simulink model "rc_update"  (R2024b)
settings: Solver=FixedStepAuto  StartTime=0.0  StopTime=10.0  FixedStep=0.005  RelTol=1e-3
undefined symbols (not defined in the file): MANUAL_CONTROL_SETPOINT, RC10_DZ, RC10_MAX, RC10_MIN, RC10_REV, RC10_TRIM, RC11_DZ, RC11_MAX, RC11_MIN, RC11_REV, RC11_TRIM, RC12_DZ, RC12_MAX, RC12_MIN, RC12_REV, RC12_TRIM, RC13_DZ, RC13_MAX, RC13_MIN, RC13_REV, RC13_TRIM, RC14_DZ, RC14_MAX, RC14_MIN, RC14_REV, RC14_TRIM, RC15_DZ, RC15_MAX, RC15_MIN, RC15_REV, RC15_TRIM, RC16_DZ, RC16_MAX, RC16_MIN, RC16_REV, RC16_TRIM, RC17_DZ, RC17_MAX, RC17_MIN, RC17_REV, RC17_TRIM, RC18_DZ, RC18_MAX, RC18_MIN, RC18_REV, RC18_TRIM, RC1_DZ, RC1_MAX, RC1_MIN, RC1_REV, RC1_TRIM, RC2_DZ, RC2_MAX, RC2_MIN, RC2_REV, RC2_TRIM, RC3_DZ, RC3_MAX, RC3_MIN, RC3_REV ... (+71)
libraries: simulink x1
settings Model: DataDictionary=nextpilot_datadict.sldd  Creator=DELL  LastModifiedBy=93114
settings OptimizationCC: DefaultUnderspecifiedDataType=single
settings DebuggingCC: UnconnectedInputMsg=warning  UnconnectedOutputMsg=warning  UnconnectedLineMsg=warning
settings ModelReferenceCC: EnableRefExpFcnMdlSchedulingChecks=on
settings RTWCC: GPUComputeCapability=3.5  DLArmComputeVersion=19.05

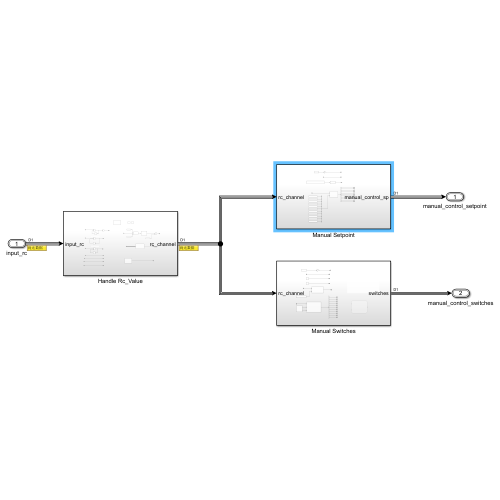
[thumbnail: Simulink's stored preview of the top-level diagram]
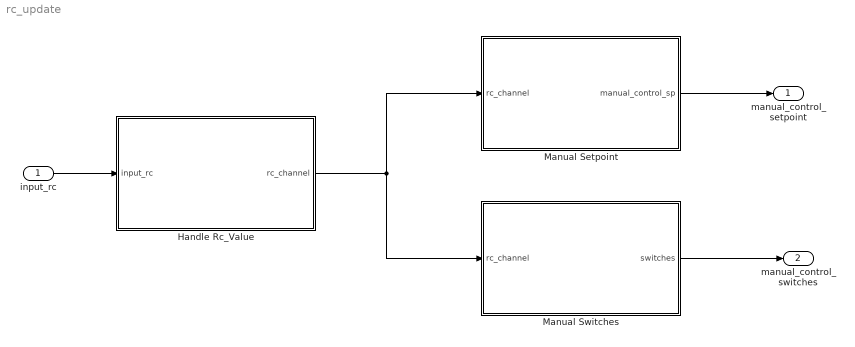
== system rc_update ==
  input_rc : Inport  OutDataTypeStr=Bus: input_rc_s
  Handle Rc_Value : Subsystem
  Manual Setpoint : Subsystem
  Manual Switches : Subsystem
  manual_control_setpoint : Outport  OutDataTypeStr=Bus: manual_control_setpoint_s
  manual_control_switches : Outport  Port=2  OutDataTypeStr=Bus: manual_control_switches_s
  wires:
  input_rc/1 -> Handle Rc_Value/1(input_rc)
  Handle Rc_Value/1(rc_channel) -> Manual Setpoint/1(rc_channel), Manual Switches/1(rc_channel)
  Manual Setpoint/1(manual_control_sp) -> manual_control_setpoint/1
  Manual Switches/1(switches) -> manual_control_switches/1

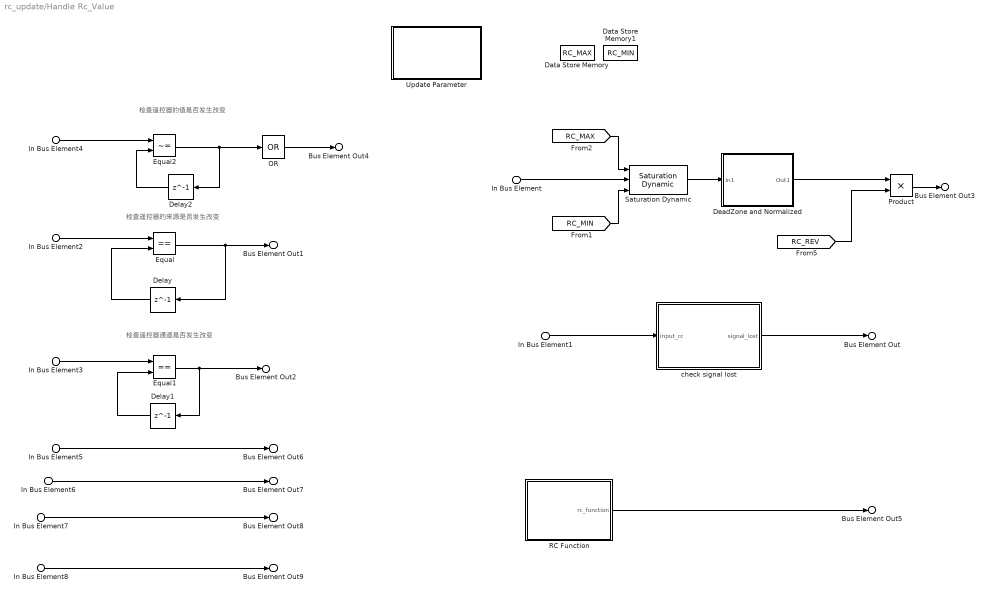
== system rc_update/Handle Rc_Value ==
  note: 检查遥控器通道是否发生改变
  note: 检查遥控器的来源是否发生改变
  note: 检查遥控器的值是否发生改变
  In Bus Element1 : Inport  PortName=input_rc
  In Bus Element : Inport  PortName=input_rc  Element=values
  In Bus Element4 : Inport  PortName=input_rc  Element=values
  In Bus Element2 : Inport  PortName=input_rc  Element=input_source
  In Bus Element3 : Inport  PortName=input_rc  Element=channel_count
  In Bus Element5 : Inport  PortName=input_rc  Element=channel_count
  In Bus Element6 : Inport  PortName=input_rc  Element=rssi
  In Bus Element7 : Inport  PortName=input_rc  Element=timestamp_last_signal
  In Bus Element8 : Inport  PortName=input_rc  Element=rc_lost_frame_count
  Data Store Memory : DataStoreMemory  DataStoreName=RC_MAX  WriteAfterWriteMsg=warning  ShowAdditionalParam=off  OutDataTypeStr=single  Dimensions=18
  Data Store Memory1 : DataStoreMemory  DataStoreName=RC_MIN  WriteAfterWriteMsg=warning  ShowAdditionalParam=off  OutDataTypeStr=single  Dimensions=18
  DeadZone and Normalized : Subsystem
  Delay : Delay  DelayLength=1
  Delay1 : Delay  DelayLength=1
  Delay2 : Delay  DelayLength=1
  Equal : RelationalOperator  Operator===  OutDataTypeStr=boolean  RndMeth=Simplest  InputSameDT=off
  Equal1 : RelationalOperator  Operator===  OutDataTypeStr=boolean  RndMeth=Simplest  InputSameDT=off
  Equal2 : RelationalOperator  Operator=~=  OutDataTypeStr=boolean  RndMeth=Simplest  InputSameDT=off
  OR : Logic  Operator=OR  Inputs=1  IconShape=distinctive  AllPortsSameDT=off  OutDataTypeStr=boolean
  Product : Product
  RC Function : Subsystem
  Saturation Dynamic : simulink/Discontinuities/Saturation Dynamic  OutMin=[]  OutMax=[]  OutDataTypeStr=Inherit: Same as second input  OutDataType=fixdt(1, 16)  OutScaling=2^-10  DoSatur=off
  Update Parameter : Subsystem
  check signal lost : Stateflow chart  TreatAsAtomicUnit=on
  Bus Element Out8 : Outport  PortName=rc_channel  Element=timestamp
  Bus Element Out3 : Outport  PortName=rc_channel  Element=channels
  Bus Element Out6 : Outport  PortName=rc_channel  Element=channel_count
  Bus Element Out5 : Outport  PortName=rc_channel  Element=function
  Bus Element Out7 : Outport  PortName=rc_channel  Element=rssi
  Bus Element Out : Outport  PortName=rc_channel  Element=signal_lost
  Bus Element Out9 : Outport  PortName=rc_channel  Element=frame_drop_count
  Bus Element Out1 : Outport  PortName=rc_channel  Element=input_source_stable
  Bus Element Out2 : Outport  PortName=rc_channel  Element=channel_count_stable
  Bus Element Out4 : Outport  PortName=rc_channel  Element=rc_updated
  wires:
  [RC_REV] -> Product/2
  Saturation Dynamic/1 -> DeadZone and Normalized/1(In1)
  DeadZone and Normalized/1(Out1) -> Product/1
  [RC_MAX] -> Saturation Dynamic/1
  [RC_MIN] -> Saturation Dynamic/3
  In Bus Element/1 -> Saturation Dynamic/2
  Product/1 -> Bus Element Out3/1
  In Bus Element1/1 -> check signal lost/1(input_rc)
  check signal lost/1(signal_lost) -> Bus Element Out/1
  In Bus Element2/1 -> Equal/1
  Equal/1 -> Bus Element Out1/1, Delay/1
  Delay/1 -> Equal/2
  In Bus Element3/1 -> Equal1/1
  Equal1/1 -> Bus Element Out2/1, Delay1/1
  Delay1/1 -> Equal1/2
  In Bus Element4/1 -> Equal2/1
  Equal2/1 -> OR/1, Delay2/1
  Delay2/1 -> Equal2/2
  OR/1 -> Bus Element Out4/1
  RC Function/1(rc_function) -> Bus Element Out5/1
  In Bus Element5/1 -> Bus Element Out6/1
  In Bus Element6/1 -> Bus Element Out7/1
  In Bus Element7/1 -> Bus Element Out8/1
  In Bus Element8/1 -> Bus Element Out9/1

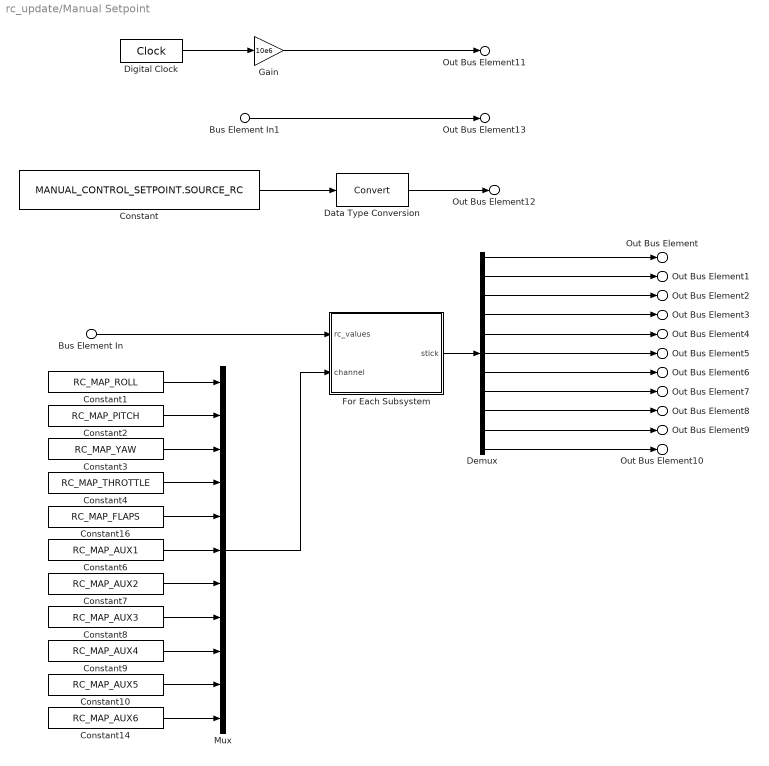
== system rc_update/Manual Setpoint ==
  Bus Element In : Inport  PortName=rc_channel  Element=channels
  Bus Element In1 : Inport  PortName=rc_channel  Element=timestamp
  Constant : Constant  Value=MANUAL_CONTROL_SETPOINT.SOURCE_RC
  Constant1 : Constant  Value=RC_MAP_ROLL
  Constant10 : Constant  Value=RC_MAP_AUX5
  Constant14 : Constant  Value=RC_MAP_AUX6
  Constant16 : Constant  Value=RC_MAP_FLAPS
  Constant2 : Constant  Value=RC_MAP_PITCH
  Constant3 : Constant  Value=RC_MAP_YAW
  Constant4 : Constant  Value=RC_MAP_THROTTLE
  Constant6 : Constant  Value=RC_MAP_AUX1
  Constant7 : Constant  Value=RC_MAP_AUX2
  Constant8 : Constant  Value=RC_MAP_AUX3
  Constant9 : Constant  Value=RC_MAP_AUX4
  Data Type Conversion : DataTypeConversion  SaturateOnIntegerOverflow=off  RndMeth=Floor
  Demux : Demux  Outputs=11.
  Digital Clock : DigitalClock  SampleTime=-1
  For Each Subsystem : Subsystem  TreatAsAtomicUnit=on
  Gain : Gain  Gain=10e6  OutDataTypeStr=uint64
  Mux : Mux  Inputs=11
  Out Bus Element11 : Outport  PortName=manual_control_sp  Element=timestamp
  Out Bus Element13 : Outport  PortName=manual_control_sp  Element=timestamp_sample
  Out Bus Element12 : Outport  PortName=manual_control_sp  Element=data_source
  Out Bus Element1 : Outport  PortName=manual_control_sp  Element=x
  Out Bus Element : Outport  PortName=manual_control_sp  Element=y
  Out Bus Element3 : Outport  PortName=manual_control_sp  Element=z
  Out Bus Element2 : Outport  PortName=manual_control_sp  Element=r
  Out Bus Element4 : Outport  PortName=manual_control_sp  Element=flaps
  Out Bus Element5 : Outport  PortName=manual_control_sp  Element=aux1
  Out Bus Element6 : Outport  PortName=manual_control_sp  Element=aux2
  Out Bus Element7 : Outport  PortName=manual_control_sp  Element=aux3
  Out Bus Element8 : Outport  PortName=manual_control_sp  Element=aux4
  Out Bus Element9 : Outport  PortName=manual_control_sp  Element=aux5
  Out Bus Element10 : Outport  PortName=manual_control_sp  Element=aux6
  wires:
  Digital Clock/1 -> Gain/1
  Constant/1 -> Data Type Conversion/1
  Bus Element In1/1 -> Out Bus Element13/1
  Gain/1 -> Out Bus Element11/1
  Data Type Conversion/1 -> Out Bus Element12/1
  Bus Element In/1 -> For Each Subsystem/1(rc_values)
  Constant1/1 -> Mux/1
  Constant2/1 -> Mux/2
  Constant4/1 -> Mux/4
  Constant3/1 -> Mux/3
  Mux/1 -> For Each Subsystem/2(channel)
  For Each Subsystem/1(stick) -> Demux/1
  Demux/5 -> Out Bus Element4/1
  Demux/4 -> Out Bus Element3/1
  Demux/6 -> Out Bus Element5/1
  Demux/3 -> Out Bus Element2/1
  Demux/7 -> Out Bus Element6/1
  Demux/2 -> Out Bus Element1/1
  Demux/8 -> Out Bus Element7/1
  Demux/1 -> Out Bus Element/1
  Demux/9 -> Out Bus Element8/1
  Demux/10 -> Out Bus Element9/1
  Demux/11 -> Out Bus Element10/1
  Constant16/1 -> Mux/5
  Constant6/1 -> Mux/6
  Constant7/1 -> Mux/7
  Constant8/1 -> Mux/8
  Constant9/1 -> Mux/9
  Constant10/1 -> Mux/10
  Constant14/1 -> Mux/11

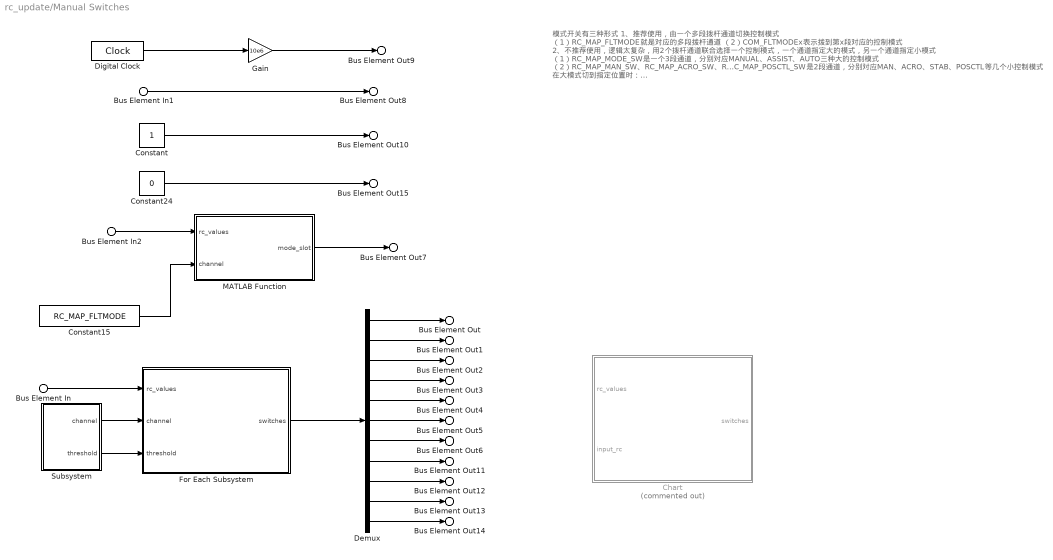
== system rc_update/Manual Switches ==
  note: 模式开关有三种形式
      |
      | 1、推荐使用，由一个多段拨杆通道切换控制模式
      | （1）RC_MAP_FLTMODE就是对应的多段拨杆通道
      | （2）COM_FLTMODEx表示拨到第x段对应的控制模式
      |
      | 2、不推荐使用，逻辑太复杂，用2个拨杆通道联合选择一个控制模式，一个通道指定大的模式，另一个通道指定小模式
      | （1）RC_MAP_MODE_SW是一个3段通道，分别对应MANUAL、ASSIST、AUTO三种大的控制模式
      | （2）RC_MAP_MAN_SW、RC_MAP_ACRO_SW、RC_MAP_STAB_SW、RC_MAP_POSCTL_SW是2段通道，分别对应MAN、ACRO、STAB、POSCTL等几个小控制模式
      |
      | 在大模式切到指定位置时：
      | （1）MANUAL模式时，优先顺序RC_MAP_MAN_SW、RC_MAP_ACRO_SW、RC_MAP_STAB_SW
      | （2）ASSIST模式时，先判断RC_MAP_POSCTL_SW通道是否打开，打开则切POSCTL，没有则切ALTCTL模式
      | （3）AUTO模式时，直接切换MISSION模式
      |
      | 3、不推荐使用，用1个按钮开关表示一个模式，长按这个按钮则切换到这个模式，
      | （1）RC_MAP_FLTM_BTN中bit位为1表示该通道作为模式按钮
      | （2）COMx_FLTMODEx表示第x个通道对应的控制模式
  Bus Element In : Inport  PortName=rc_channel  Element=channels
  Bus Element In2 : Inport  PortName=rc_channel  Element=channels
  Bus Element In1 : Inport  PortName=rc_channel  Element=timestamp
  Chart : Stateflow chart  Commented=on  TreatAsAtomicUnit=on
  Constant : Constant  OutDataTypeStr=uint32
  Constant15 : Constant  Value=RC_MAP_FLTMODE  OutDataTypeStr=single
  Constant24 : Constant  Value=0  OutDataTypeStr=uint8
  Demux : Demux  Outputs=11
  Digital Clock : DigitalClock  SampleTime=-1
  For Each Subsystem : Subsystem  TreatAsAtomicUnit=on
  Gain : Gain  Gain=10e6  OutDataTypeStr=uint64
  MATLAB Function : MATLAB Function  TreatAsAtomicUnit=on
  Subsystem : Subsystem
  Bus Element Out9 : Outport  PortName=switches  Element=timestamp
  Bus Element Out8 : Outport  PortName=switches  Element=timestamp_sample
  Bus Element Out7 : Outport  PortName=switches  Element=mode_slot
  Bus Element Out4 : Outport  PortName=switches  Element=arm_switch
  Bus Element Out : Outport  PortName=switches  Element=return_switch
  Bus Element Out1 : Outport  PortName=switches  Element=loiter_switch
  Bus Element Out2 : Outport  PortName=switches  Element=offboard_switch
  Bus Element Out3 : Outport  PortName=switches  Element=kill_switch
  Bus Element Out6 : Outport  PortName=switches  Element=gear_switch
  Bus Element Out5 : Outport  PortName=switches  Element=transition_switch
  Bus Element Out15 : Outport  PortName=switches  Element=mode_switch
  Bus Element Out11 : Outport  PortName=switches  Element=man_switch
  Bus Element Out12 : Outport  PortName=switches  Element=acro_switch
  Bus Element Out13 : Outport  PortName=switches  Element=stab_switch
  Bus Element Out14 : Outport  PortName=switches  Element=posctl_switch
  Bus Element Out10 : Outport  PortName=switches  Element=switch_changes
  wires:
  Demux/1 -> Bus Element Out/1
  Demux/2 -> Bus Element Out1/1
  Demux/3 -> Bus Element Out2/1
  Demux/4 -> Bus Element Out3/1
  Demux/5 -> Bus Element Out4/1
  Demux/6 -> Bus Element Out5/1
  Demux/7 -> Bus Element Out6/1
  Constant15/1 -> MATLAB Function/2(channel)
  Bus Element In2/1 -> MATLAB Function/1(rc_values)
  MATLAB Function/1(mode_slot) -> Bus Element Out7/1
  Bus Element In1/1 -> Bus Element Out8/1
  Gain/1 -> Bus Element Out9/1
  Digital Clock/1 -> Gain/1
  Constant/1 -> Bus Element Out10/1
  For Each Subsystem/1(switches) -> Demux/1
  Demux/8 -> Bus Element Out11/1
  Demux/9 -> Bus Element Out12/1
  Demux/10 -> Bus Element Out13/1
  Demux/11 -> Bus Element Out14/1
  Constant24/1 -> Bus Element Out15/1
  Bus Element In/1 -> For Each Subsystem/1(rc_values)
  Subsystem/1(channel) -> For Each Subsystem/2(channel)
  Subsystem/2(threshold) -> For Each Subsystem/3(threshold)

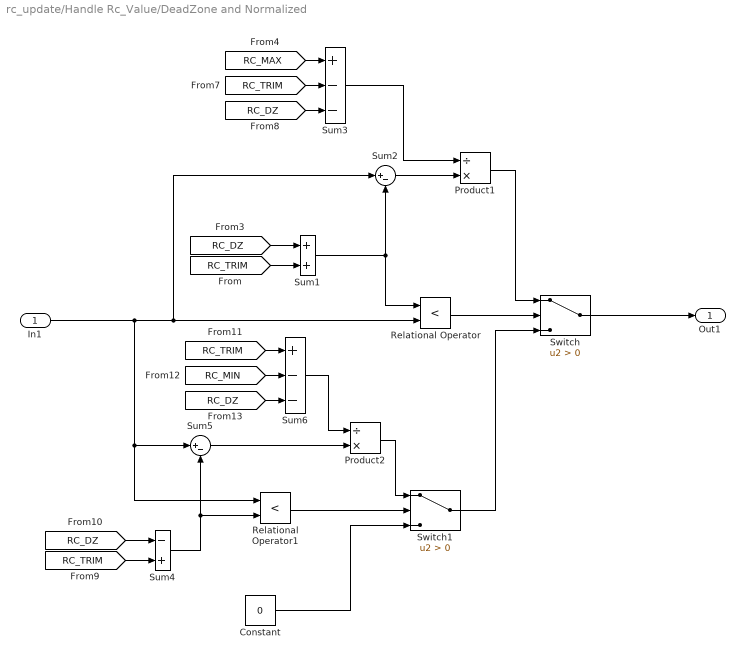
== system rc_update/Handle Rc_Value/DeadZone and Normalized ==
  In1 : Inport
  Constant : Constant  Value=0  OutDataTypeStr=single
  Product1 : Product  Inputs=/*
  Product2 : Product  Inputs=/*
  Relational Operator : RelationalOperator  Operator=<  OutDataTypeStr=boolean  RndMeth=Simplest  InputSameDT=off
  Relational Operator1 : RelationalOperator  Operator=<  OutDataTypeStr=boolean  RndMeth=Simplest  InputSameDT=off
  Sum1 : Sum  Inputs=2
  Sum2 : Sum  Inputs=|+-
  Sum3 : Sum  Inputs=+--
  Sum4 : Sum  Inputs=-+
  Sum5 : Sum  Inputs=|+-
  Sum6 : Sum  Inputs=+--
  Switch : Switch  Criteria=u2 > Threshold  SaturateOnIntegerOverflow=off  InputSameDT=off
  Switch1 : Switch  Criteria=u2 > Threshold  SaturateOnIntegerOverflow=off  InputSameDT=off
  Out1 : Outport
  wires:
  [RC_MAX] -> Sum3/1
  Sum3/1 -> Product1/1
  Product2/1 -> Switch1/1
  [RC_TRIM] -> Sum1/2
  [RC_DZ] -> Sum6/3
  Sum1/1 -> Relational Operator/1, Sum2/2
  [RC_TRIM] -> Sum3/2
  Relational Operator1/1 -> Switch1/2
  In1/1 -> Sum5/1, Relational Operator1/1, Sum2/1, Relational Operator/2
  Sum5/1 -> Product2/2
  Sum4/1 -> Sum5/2, Relational Operator1/2
  [RC_DZ] -> Sum3/3
  [RC_DZ] -> Sum1/1
  Sum2/1 -> Product1/2
  [RC_DZ] -> Sum4/1
  [RC_TRIM] -> Sum4/2
  Switch1/1 -> Switch/3
  Constant/1 -> Switch1/3
  [RC_MIN] -> Sum6/2
  Sum6/1 -> Product2/1
  Product1/1 -> Switch/1
  Relational Operator/1 -> Switch/2
  [RC_TRIM] -> Sum6/1
  Switch/1 -> Out1/1

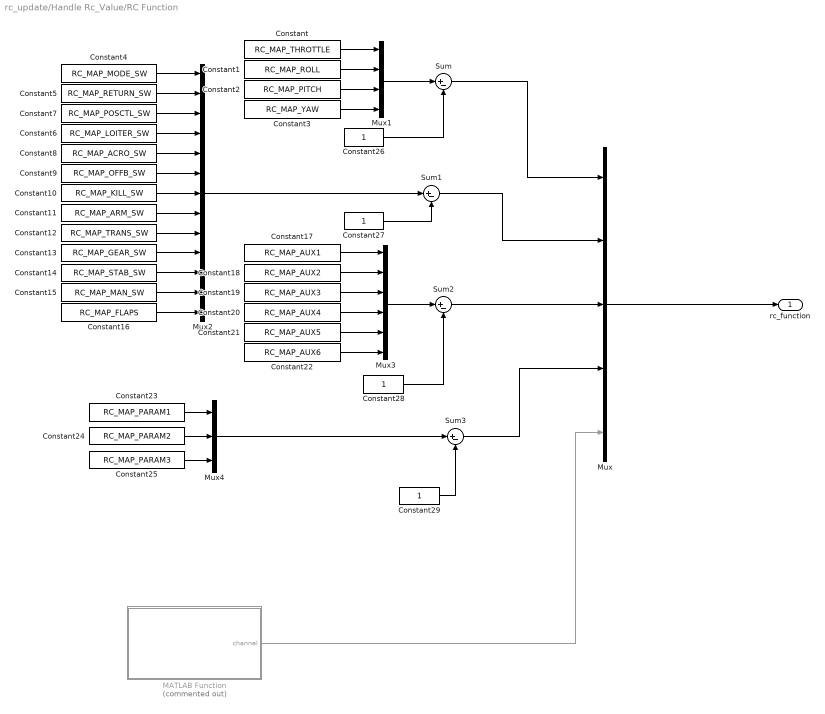
== system rc_update/Handle Rc_Value/RC Function ==
  Constant : Constant  Value=RC_MAP_THROTTLE
  Constant1 : Constant  Value=RC_MAP_ROLL
  Constant10 : Constant  Value=RC_MAP_KILL_SW
  Constant11 : Constant  Value=RC_MAP_ARM_SW
  Constant12 : Constant  Value=RC_MAP_TRANS_SW
  Constant13 : Constant  Value=RC_MAP_GEAR_SW
  Constant14 : Constant  Value=RC_MAP_STAB_SW
  Constant15 : Constant  Value=RC_MAP_MAN_SW
  Constant16 : Constant  Value=RC_MAP_FLAPS
  Constant17 : Constant  Value=RC_MAP_AUX1
  Constant18 : Constant  Value=RC_MAP_AUX2
  Constant19 : Constant  Value=RC_MAP_AUX3
  Constant2 : Constant  Value=RC_MAP_PITCH
  Constant20 : Constant  Value=RC_MAP_AUX4
  Constant21 : Constant  Value=RC_MAP_AUX5
  Constant22 : Constant  Value=RC_MAP_AUX6
  Constant23 : Constant  Value=RC_MAP_PARAM1
  Constant24 : Constant  Value=RC_MAP_PARAM2
  Constant25 : Constant  Value=RC_MAP_PARAM3
  Constant{26..29} (4 alike) : Constant  OutDataTypeStr=int8
  Constant3 : Constant  Value=RC_MAP_YAW
  Constant4 : Constant  Value=RC_MAP_MODE_SW
  Constant5 : Constant  Value=RC_MAP_RETURN_SW
  Constant6 : Constant  Value=RC_MAP_LOITER_SW
  Constant7 : Constant  Value=RC_MAP_POSCTL_SW
  Constant8 : Constant  Value=RC_MAP_ACRO_SW
  Constant9 : Constant  Value=RC_MAP_OFFB_SW
  MATLAB Function : MATLAB Function  Commented=on  TreatAsAtomicUnit=on
  Mux : Mux  Inputs=5
  Mux1 : Mux
  Mux2 : Mux  Inputs=13
  Mux3 : Mux  Inputs=6
  Mux4 : Mux  Inputs=3
  Sum{,1..3} (4 alike) : Sum  Inputs=|+-  OutDataTypeStr=int8
  rc_function : Outport
  wires:
  Mux/1 -> rc_function/1
  Constant2/1 -> Mux1/3
  Constant1/1 -> Mux1/2
  Constant/1 -> Mux1/1
  Constant3/1 -> Mux1/4
  Constant4/1 -> Mux2/1
  Constant5/1 -> Mux2/2
  Constant7/1 -> Mux2/3
  Constant6/1 -> Mux2/4
  Constant11/1 -> Mux2/8
  Constant12/1 -> Mux2/9
  Constant13/1 -> Mux2/10
  Constant14/1 -> Mux2/11
  Constant15/1 -> Mux2/12
  Constant16/1 -> Mux2/13
  Constant8/1 -> Mux2/5
  Constant9/1 -> Mux2/6
  Constant10/1 -> Mux2/7
  Constant17/1 -> Mux3/1
  Constant18/1 -> Mux3/2
  Constant19/1 -> Mux3/3
  Constant20/1 -> Mux3/4
  Constant21/1 -> Mux3/5
  Constant22/1 -> Mux3/6
  Constant23/1 -> Mux4/1
  Constant24/1 -> Mux4/2
  Constant25/1 -> Mux4/3
  Mux4/1 -> Sum3/1
  MATLAB Function/1(channel) -> Mux/5
  Mux1/1 -> Sum/1
  Sum/1 -> Mux/1
  Constant26/1 -> Sum/2
  Mux2/1 -> Sum1/1
  Constant27/1 -> Sum1/2
  Sum1/1 -> Mux/2
  Mux3/1 -> Sum2/1
  Sum2/1 -> Mux/3
  Constant28/1 -> Sum2/2
  Constant29/1 -> Sum3/2
  Sum3/1 -> Mux/4

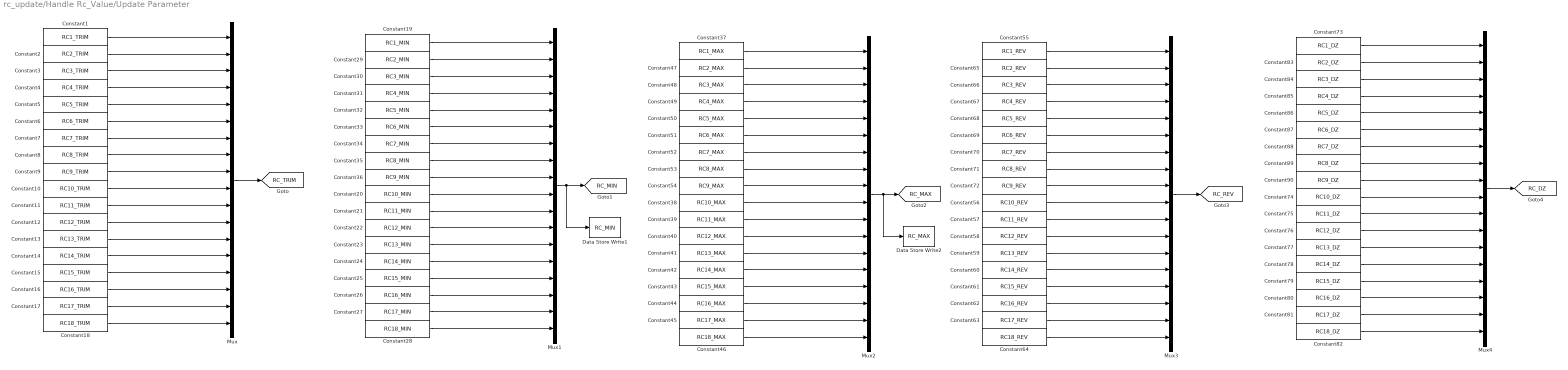
== system rc_update/Handle Rc_Value/Update Parameter ==
  Constant1 : Constant  Value=RC1_TRIM
  Constant10 : Constant  Value=RC10_TRIM
  Constant11 : Constant  Value=RC11_TRIM
  Constant12 : Constant  Value=RC12_TRIM
  Constant13 : Constant  Value=RC13_TRIM
  Constant14 : Constant  Value=RC14_TRIM
  Constant15 : Constant  Value=RC15_TRIM
  Constant16 : Constant  Value=RC16_TRIM
  Constant17 : Constant  Value=RC17_TRIM
  Constant18 : Constant  Value=RC18_TRIM
  Constant19 : Constant  Value=RC1_MIN
  Constant2 : Constant  Value=RC2_TRIM
  Constant20 : Constant  Value=RC10_MIN
  Constant21 : Constant  Value=RC11_MIN
  Constant22 : Constant  Value=RC12_MIN
  Constant23 : Constant  Value=RC13_MIN
  Constant24 : Constant  Value=RC14_MIN
  Constant25 : Constant  Value=RC15_MIN
  Constant26 : Constant  Value=RC16_MIN
  Constant27 : Constant  Value=RC17_MIN
  Constant28 : Constant  Value=RC18_MIN
  Constant29 : Constant  Value=RC2_MIN
  Constant3 : Constant  Value=RC3_TRIM
  Constant30 : Constant  Value=RC3_MIN
  Constant31 : Constant  Value=RC4_MIN
  Constant32 : Constant  Value=RC5_MIN
  Constant33 : Constant  Value=RC6_MIN
  Constant34 : Constant  Value=RC7_MIN
  Constant35 : Constant  Value=RC8_MIN
  Constant36 : Constant  Value=RC9_MIN
  Constant37 : Constant  Value=RC1_MAX
  Constant38 : Constant  Value=RC10_MAX
  Constant39 : Constant  Value=RC11_MAX
  Constant4 : Constant  Value=RC4_TRIM
  Constant40 : Constant  Value=RC12_MAX
  Constant41 : Constant  Value=RC13_MAX
  Constant42 : Constant  Value=RC14_MAX
  Constant43 : Constant  Value=RC15_MAX
  Constant44 : Constant  Value=RC16_MAX
  Constant45 : Constant  Value=RC17_MAX
  Constant46 : Constant  Value=RC18_MAX
  Constant47 : Constant  Value=RC2_MAX
  Constant48 : Constant  Value=RC3_MAX
  Constant49 : Constant  Value=RC4_MAX
  Constant5 : Constant  Value=RC5_TRIM
  Constant50 : Constant  Value=RC5_MAX
  Constant51 : Constant  Value=RC6_MAX
  Constant52 : Constant  Value=RC7_MAX
  Constant53 : Constant  Value=RC8_MAX
  Constant54 : Constant  Value=RC9_MAX
  Constant55 : Constant  Value=RC1_REV
  Constant56 : Constant  Value=RC10_REV
  Constant57 : Constant  Value=RC11_REV
  Constant58 : Constant  Value=RC12_REV
  Constant59 : Constant  Value=RC13_REV
  Constant6 : Constant  Value=RC6_TRIM
  Constant60 : Constant  Value=RC14_REV
  Constant61 : Constant  Value=RC15_REV
  Constant62 : Constant  Value=RC16_REV
  Constant63 : Constant  Value=RC17_REV
  Constant64 : Constant  Value=RC18_REV
  Constant65 : Constant  Value=RC2_REV
  Constant66 : Constant  Value=RC3_REV
  Constant67 : Constant  Value=RC4_REV
  Constant68 : Constant  Value=RC5_REV
  Constant69 : Constant  Value=RC6_REV
  Constant7 : Constant  Value=RC7_TRIM
  Constant70 : Constant  Value=RC7_REV
  Constant71 : Constant  Value=RC8_REV
  Constant72 : Constant  Value=RC9_REV
  Constant73 : Constant  Value=RC1_DZ
  Constant74 : Constant  Value=RC10_DZ
  Constant75 : Constant  Value=RC11_DZ
  Constant76 : Constant  Value=RC12_DZ
  Constant77 : Constant  Value=RC13_DZ
  Constant78 : Constant  Value=RC14_DZ
  Constant79 : Constant  Value=RC15_DZ
  Constant8 : Constant  Value=RC8_TRIM
  Constant80 : Constant  Value=RC16_DZ
  Constant81 : Constant  Value=RC17_DZ
  Constant82 : Constant  Value=RC18_DZ
  Constant83 : Constant  Value=RC2_DZ
  Constant84 : Constant  Value=RC3_DZ
  Constant85 : Constant  Value=RC4_DZ
  Constant86 : Constant  Value=RC5_DZ
  Constant87 : Constant  Value=RC6_DZ
  Constant88 : Constant  Value=RC7_DZ
  Constant89 : Constant  Value=RC8_DZ
  Constant9 : Constant  Value=RC9_TRIM
  Constant90 : Constant  Value=RC9_DZ
  Data Store Write1 : DataStoreWrite  DataStoreName=RC_MIN  IndexOptions=Index vector (dialog)  Indices=1  OutputSizes=1
  Data Store Write2 : DataStoreWrite  DataStoreName=RC_MAX  IndexOptions=Index vector (dialog)  Indices=1  OutputSizes=1
  Mux{,1..4} (5 alike) : Mux  Inputs=18
  tag scope: RC_DZ=global, RC_MAX=global, RC_MIN=global, RC_REV=global, RC_TRIM=global
  wires:
  Constant3/1 -> Mux/3
  Constant12/1 -> Mux/12
  Constant13/1 -> Mux/13
  Constant10/1 -> Mux/10
  Constant1/1 -> Mux/1
  Constant2/1 -> Mux/2
  Constant18/1 -> Mux/18
  Constant11/1 -> Mux/11
  Constant4/1 -> Mux/4
  Constant5/1 -> Mux/5
  Constant6/1 -> Mux/6
  Constant17/1 -> Mux/17
  Constant7/1 -> Mux/7
  Constant14/1 -> Mux/14
  Constant8/1 -> Mux/8
  Constant9/1 -> Mux/9
  Constant15/1 -> Mux/15
  Constant16/1 -> Mux/16
  Mux/1 -> [RC_TRIM]
  Constant26/1 -> Mux1/16
  Constant25/1 -> Mux1/15
  Constant36/1 -> Mux1/9
  Constant35/1 -> Mux1/8
  Constant32/1 -> Mux1/5
  Constant33/1 -> Mux1/6
  Constant27/1 -> Mux1/17
  Constant34/1 -> Mux1/7
  Constant24/1 -> Mux1/14
  Constant31/1 -> Mux1/4
  Constant21/1 -> Mux1/11
  Constant19/1 -> Mux1/1
  Constant23/1 -> Mux1/13
  Constant20/1 -> Mux1/10
  Constant22/1 -> Mux1/12
  Constant30/1 -> Mux1/3
  Constant28/1 -> Mux1/18
  Constant29/1 -> Mux1/2
  Mux1/1 -> Data Store Write1/1, [RC_MIN]
  Constant44/1 -> Mux2/16
  Mux2/1 -> Data Store Write2/1, [RC_MAX]
  Constant47/1 -> Mux2/2
  Constant48/1 -> Mux2/3
  Constant46/1 -> Mux2/18
  Constant40/1 -> Mux2/12
  Constant37/1 -> Mux2/1
  Constant39/1 -> Mux2/11
  Constant41/1 -> Mux2/13
  Constant52/1 -> Mux2/7
  Constant51/1 -> Mux2/6
  Constant38/1 -> Mux2/10
  Constant45/1 -> Mux2/17
  Constant49/1 -> Mux2/4
  Constant50/1 -> Mux2/5
  Constant43/1 -> Mux2/15
  Constant53/1 -> Mux2/8
  Constant54/1 -> Mux2/9
  Constant42/1 -> Mux2/14
  Constant67/1 -> Mux3/4
  Constant63/1 -> Mux3/17
  Constant60/1 -> Mux3/14
  Constant72/1 -> Mux3/9
  Constant68/1 -> Mux3/5
  Constant61/1 -> Mux3/15
  Constant71/1 -> Mux3/8
  Constant70/1 -> Mux3/7
  Constant56/1 -> Mux3/10
  Constant69/1 -> Mux3/6
  Constant59/1 -> Mux3/13
  Constant57/1 -> Mux3/11
  Constant55/1 -> Mux3/1
  Constant65/1 -> Mux3/2
  Mux3/1 -> [RC_REV]
  Constant58/1 -> Mux3/12
  Constant62/1 -> Mux3/16
  Constant66/1 -> Mux3/3
  Constant64/1 -> Mux3/18
  Constant82/1 -> Mux4/18
  Mux4/1 -> [RC_DZ]
  Constant84/1 -> Mux4/3
  Constant80/1 -> Mux4/16
  Constant76/1 -> Mux4/12
  Constant73/1 -> Mux4/1
  Constant75/1 -> Mux4/11
  Constant77/1 -> Mux4/13
  Constant87/1 -> Mux4/6
  Constant83/1 -> Mux4/2
  Constant88/1 -> Mux4/7
  Constant90/1 -> Mux4/9
  Constant86/1 -> Mux4/5
  Constant79/1 -> Mux4/15
  Constant78/1 -> Mux4/14
  Constant74/1 -> Mux4/10
  Constant89/1 -> Mux4/8
  Constant81/1 -> Mux4/17
  Constant85/1 -> Mux4/4

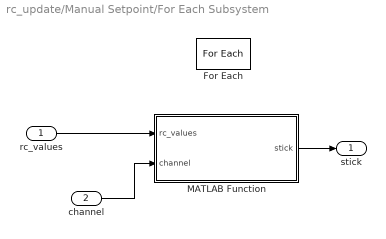
== system rc_update/Manual Setpoint/For Each Subsystem ==
  rc_values : Inport
  channel : Inport  Port=2  Partition=on  PartitionDimension=1  PartitionWidth=1  PartitionOffset=0
  For Each : ForEach  DisableCoverage=on
  MATLAB Function : MATLAB Function  TreatAsAtomicUnit=on
  stick : Outport  ConcatenationDimension=1
  wires:
  rc_values/1 -> MATLAB Function/1(rc_values)
  channel/1 -> MATLAB Function/2(channel)
  MATLAB Function/1(stick) -> stick/1

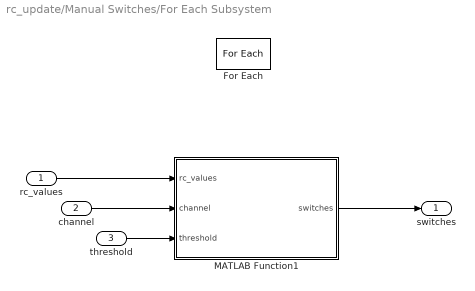
== system rc_update/Manual Switches/For Each Subsystem ==
  rc_values : Inport
  channel : Inport  Port=2  Partition=on  PartitionDimension=1  PartitionWidth=1  PartitionOffset=0
  threshold : Inport  Port=3  Partition=on  PartitionDimension=1  PartitionWidth=1  PartitionOffset=0
  For Each : ForEach  DisableCoverage=on
  MATLAB Function1 : MATLAB Function  TreatAsAtomicUnit=on
  switches : Outport  ConcatenationDimension=1
  wires:
  MATLAB Function1/1(switches) -> switches/1
  rc_values/1 -> MATLAB Function1/1(rc_values)
  channel/1 -> MATLAB Function1/2(channel)
  threshold/1 -> MATLAB Function1/3(threshold)

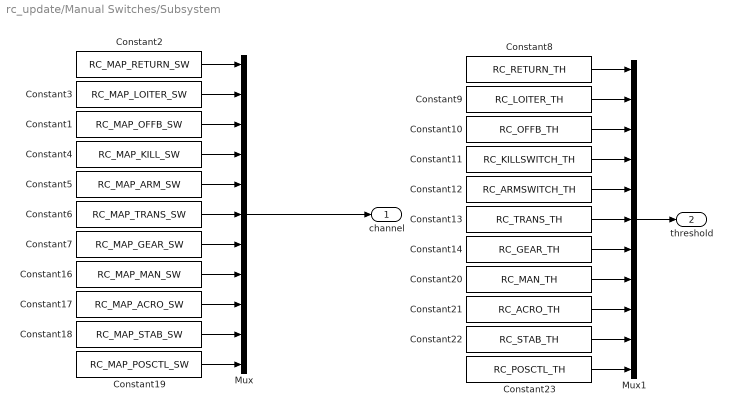
== system rc_update/Manual Switches/Subsystem ==
  Constant1 : Constant  Value=RC_MAP_OFFB_SW  OutDataTypeStr=single
  Constant10 : Constant  Value=RC_OFFB_TH  OutDataTypeStr=single
  Constant11 : Constant  Value=RC_KILLSWITCH_TH  OutDataTypeStr=single
  Constant12 : Constant  Value=RC_ARMSWITCH_TH  OutDataTypeStr=single
  Constant13 : Constant  Value=RC_TRANS_TH  OutDataTypeStr=single
  Constant14 : Constant  Value=RC_GEAR_TH  OutDataTypeStr=single
  Constant16 : Constant  Value=RC_MAP_MAN_SW  OutDataTypeStr=single
  Constant17 : Constant  Value=RC_MAP_ACRO_SW  OutDataTypeStr=single
  Constant18 : Constant  Value=RC_MAP_STAB_SW  OutDataTypeStr=single
  Constant19 : Constant  Value=RC_MAP_POSCTL_SW  OutDataTypeStr=single
  Constant2 : Constant  Value=RC_MAP_RETURN_SW  OutDataTypeStr=single
  Constant20 : Constant  Value=RC_MAN_TH  OutDataTypeStr=single
  Constant21 : Constant  Value=RC_ACRO_TH  OutDataTypeStr=single
  Constant22 : Constant  Value=RC_STAB_TH  OutDataTypeStr=single
  Constant23 : Constant  Value=RC_POSCTL_TH  OutDataTypeStr=single
  Constant3 : Constant  Value=RC_MAP_LOITER_SW  OutDataTypeStr=single
  Constant4 : Constant  Value=RC_MAP_KILL_SW  OutDataTypeStr=single
  Constant5 : Constant  Value=RC_MAP_ARM_SW  OutDataTypeStr=single
  Constant6 : Constant  Value=RC_MAP_TRANS_SW  OutDataTypeStr=single
  Constant7 : Constant  Value=RC_MAP_GEAR_SW  OutDataTypeStr=single
  Constant8 : Constant  Value=RC_RETURN_TH  OutDataTypeStr=single
  Constant9 : Constant  Value=RC_LOITER_TH  OutDataTypeStr=single
  Mux : Mux  Inputs=11.
  Mux1 : Mux  Inputs=11
  channel : Outport
  threshold : Outport  Port=2
  wires:
  Constant2/1 -> Mux/1
  Constant6/1 -> Mux/6
  Constant17/1 -> Mux/9
  Constant7/1 -> Mux/7
  Constant5/1 -> Mux/5
  Constant4/1 -> Mux/4
  Constant1/1 -> Mux/3
  Constant3/1 -> Mux/2
  Constant19/1 -> Mux/11
  Constant18/1 -> Mux/10
  Constant16/1 -> Mux/8
  Mux/1 -> channel/1
  Constant23/1 -> Mux1/11
  Constant22/1 -> Mux1/10
  Constant20/1 -> Mux1/8
  Constant13/1 -> Mux1/6
  Constant9/1 -> Mux1/2
  Constant12/1 -> Mux1/5
  Constant11/1 -> Mux1/4
  Constant10/1 -> Mux1/3
  Constant14/1 -> Mux1/7
  Constant21/1 -> Mux1/9
  Constant8/1 -> Mux1/1
  Mux1/1 -> threshold/1

== stateflow chart rc_update/Manual Switches/Chart ==
  note: 推荐使用
      | 该方式，由一个多段拨杆通道切换控制模式
      | （1）RC_MAP_FLTMODE就是对应的多段拨杆通道
      | （2）COM_FLTMODEx表示拨到第x段对应的控制模式
  note: 不推荐使用，逻辑太复杂
      | 该方式，用2个拨杆通道联合选择一个控制模式，一个通道指定大的模式，另一个通道指定小模式
      | （1）RC_MAP_MODE_SW是一个3段通道，分别对应MANUAL、ASSIST、AUTO三种大的控制模式
      | （2）RC_MAP_MAN_SW、RC_MAP_ACRO_SW、RC_MAP_STAB_SW、RC_MAP_POSCTL_SW是2段通道，分别对应MAN、ACRO、STAB、POSCTL等几个小控制模式
      |
      | 在大模式切到指定位置时：
      | （1）MANUAL模式时，优先顺序RC_MAP_MAN_SW、RC_MAP_ACRO_SW、RC_MAP_STAB_SW
      | （2）ASSIST模式时，先判断RC_MAP_POSCTL_SW通道是否打开，打开则切POSCTL，没有则切ALTCTL模式
      | （3）AUTO模式时，直接切换MISSION模式
  note: 该方式，用1个按钮开关表示一个模式，长按这个按钮则切换到这个模式，
      | （1）RC_MAP_FLTM_BTN指定哪几个通道作为按钮开关
      | （2）COMx_FLTMODEx表示第x个通道对应的控制模式
  note: RC_MAP_POSCTL_SW
  (default) -> (junction 7)
  (junction 20) -> (junction 21) : {
      | num_slots = uint8(PX4_MANUAL_CONTROL_SWITCHES.MODE_SLOT_NUM);
      | slot_width_half  = single(1) / single(num_slots);
      | slot_min = single(-1.05);
      | slot_max = single(1.05);
      | value = rc_values(RC_MAP_FLTMODE);
      | mode_slot = floor((((((value - slot_min) * single(num_slots)) + slot_width_half) / (slot_max - slot_min)) + slot_width_half) + 1.0);
      | switches.mode_slot = min(num_slots, uint8(mode_slot));
      | }
  (junction 7) -> (junction 20) [order 1] : [RC_MAP_FLTMODE > 0]
  (junction 21) -> (junction 23)
  (junction 7) -> (junction 16) [order 2]
  (junction 18) -> (junction 23) : {
      | switches.mode_switch = get_rc_sw3pos_position(RC_MAP_MODE_SW, RC_AUTO_TH, RC_ASSIST_TH);
      | switches.man_switch = get_rc_sw2pos_position(RC_MAP_MAN_SW, RC_MAN_TH);
      | switches.acro_switch = get_rc_sw2pos_position(RC_MAP_ACRO_SW, RC_ACRO_TH);
      | switches.stab_switch = get_rc_sw2pos_position(RC_MAP_STAB_SW, RC_STAB_TH);
      | switches.posctl_switch = get_rc_sw2pos_position(RC_MAP_POSCTL_SW, RC_POSCTL_TH);
      | }
  (junction 16) -> (junction 18) [order 1] : [RC_MAP_MODE_SW >0]
  (junction 23) -> (junction 30)
  (junction 16) -> (junction 26) [order 2]
  (junction 57) -> (junction 59) : {switches.mode_slot = slotpressed;}
  (junction 55) -> (junction 57) [order 1] : [duration(ispressed, usec) >50]
  (junction 59) -> (junction 30)
  (junction 26) -> (junction 28) [order 1] : [RC_MAP_FLTM_BTN > 0]
  (junction 28) -> (junction 55) : {
      | [ispressed, slotpressed] = get_rc_fltmode_button();
      | switches.mode_slot = uint8(0);
      | }
  (junction 64) -> (junction 30)
  (junction 55) -> (junction 62) [order 2]
  (junction 30) -> (junction 33)
  (junction 26) -> (junction 35) [order 2]
  (junction 62) -> (junction 64)
  (junction 33) -> (junction 35)
  (junction 35) -> (junction 9) : {
      | switches.return_switch = get_rc_sw2pos_position(RC_MAP_RETURN_SW, RC_RETURN_TH);
      | switches.loiter_switch = get_rc_sw2pos_position(RC_MAP_LOITER_SW, RC_LOITER_TH);
      | switches.offboard_switch = get_rc_sw2pos_position(RC_MAP_OFFB_SW, RC_OFFB_TH);
      | switches.kill_switch = get_rc_sw2pos_position(RC_MAP_KILL_SW, RC_KILLSWITCH_TH);
      | switches.arm_switch = get_rc_sw2pos_position(RC_MAP_ARM_SW, RC_ARMSWITCH_TH);
      | switches.transition_switch = get_rc_sw2pos_position(RC_MAP_TRANS_SW, RC_TRANS_TH);
      | switches.gear_switch = get_rc_sw2pos_position(RC_MAP_GEAR_SW, RC_GEAR_TH);
      | }
  (junction 9) -> (junction 46) : {
      | switches.timestamp = hrt_absolute_time();
      | switches.timestamp_sample = last_switches_updated_time;
      | last_switches_updated_time = switches.timestamp;
      | }
  data: chan function_input; on_th function_input; pos function_output; chan function_input; on_th function_input; pos function_output; mid_th function_input; is_consistent_button_press function_output; slot function_output; rc_values input; input_rc input; switches output Bus: px4_manual_control_switches size=1; RC_MAP_RETURN_SW parameter; RC_RETURN_TH parameter; slotpressed local; slot_max local; value local; slot_min local; last_switches_updated_time local =uint64(0); ispressed local =false; num_slots local; slot_width_half local; mode_slot local; RC_MAP_TRANS_SW parameter; RC_MAP_KILL_SW parameter; RC_KILLSWITCH_TH parameter; RC_MAP_ARM_SW parameter; RC_ARMSWITCH_TH parameter; RC_MAP_GEAR_SW parameter; RC_GEAR_TH parameter; RC_TRANS_TH parameter; RC_MAP_FLTM_BTN parameter; RC_MAP_OFFB_SW parameter; RC_MAP_LOITER_SW parameter; RC_LOITER_TH parameter; RC_OFFB_TH parameter; RC_MAP_FLTMODE parameter; RC_MAP_MAN_SW parameter; RC_MAP_POSCTL_SW parameter; RC_MAN_TH parameter; RC_AUTO_TH parameter; RC_ASSIST_TH parameter; RC_MAP_STAB_SW parameter; RC_MAP_MODE_SW parameter; RC_STAB_TH parameter; RC_ACRO_TH parameter; RC_POSCTL_TH parameter; RC_MAP_ACRO_SW parameter; RC_MAP_FLIGHT_MODE_BUTTONS data_store_memory
  function pos = get_rc_sw2pos_position(chan, on_th):
    | function pos = get_rc_sw2pos_position(chan, on_th)
    | 
    | if (chan > 0)
    |     on_inv = on_th < 0.0;
    |     value = 0.5 * rc_values(chan) + 0.5;
    |     if on_inv && value < on_th || ~on_inv && value > on_th
    |         pos = uint8(PX4_MANUAL_CONTROL_SWITCHES.SWITCH_POS_ON);
    |     else
    |         pos = uint8(PX4_MANUAL_CONTROL_SWITCHES.SWITCH_POS_OFF);
    |     end
    | else
    |     pos = uint8(PX4_MANUAL_CONTROL_SWITCHES.SWITCH_POS_NONE);
    | end
  function pos = get_rc_sw3pos_position(chan, on_th, mid_th):
    | function pos = get_rc_sw3pos_position(chan, on_th, mid_th)
    | 
    | if (chan > 0)
    |     on_inv = on_th < 0.0;
    |     mid_inv = mid_th < 0.0;
    |     value = 0.5 * rc_values(chan) + 0.5;
    |     if on_inv && value < on_th || ~on_inv && value > on_th
    |         pos = uint8(PX4_MANUAL_CONTROL_SWITCHES.SWITCH_POS_ON);
    |     elseif mid_inv && value < mid_th || ~mid_inv && value > mid_th
    |         pos = uint8(PX4_MANUAL_CONTROL_SWITCHES.SWITCH_POS_MIDDLE);
    |     else
    |         pos = uint8(PX4_MANUAL_CONTROL_SWITCHES.SWITCH_POS_OFF);
    |     end
    | else
    |     pos = uint8(PX4_MANUAL_CONTROL_SWITCHES.SWITCH_POS_NONE);
    | end
  function [is_consistent_button_press,slot]= get_rc_fltmode_button:
    | function [is_consistent_button_press,slot]= get_rc_fltmode_button()
    | persistent potential_button_press_slot;
    | if isempty(potential_button_press_slot)
    |     potential_button_press_slot = uint8(0);
    | end
    | 
    | 
    | is_consistent_button_press = false;
    | 
    | for slot = uint8(1):uint8(6)
    |     value = rc_values(RC_MAP_FLIGHT_MODE_BUTTONS(slot));
    |     if value > 0.5
    |         if slot == potential_button_press_slot
    |             is_consistent_button_press = true;
    |         end
    |         potential_button_press_slot = slot;
    |         break;
    |     end
    | end

== stateflow chart rc_update/Handle Rc_Value/check signal lost ==
  state rfd_rc_lost_check [function]
    (default) -> (junction 216)
    (junction 216) -> (junction 219) : {index=1;}
    (junction 217) -> (junction 218) [order 1] : [index <= 12 && ...
        | input_rc.values(index) > 999 && ...
        | input_rc.values(index) < 1005]
    (junction 219) -> (junction 217) [order 1] : [index<=16]
    (junction 217) -> (junction 220) [order 2]
    (junction 218) -> (junction 224) : {signal_lost=true;}
    (junction 222) -> (junction 219) : {index=index+1;}
    (junction 219) -> (junction 225) [order 2]
    (junction 220) -> (junction 221) [order 1] : [input_rc.values(index)==0]
    (junction 220) -> (junction 222) [order 2] : {signal_lost= false;}
    (junction 221) -> (junction 223) : {signal_lost= true;}
    (junction 223) -> (junction 222)
    (junction 224) -> (junction 223)
  state failsafe_rc_lost_check [function]
    (default) -> (junction 189) : {signal_lost= false;}
    (junction 189) -> (junction 190) [order 1] : [RC_MAP_FAILSAFE > 0]
    (junction 189) -> (junction 191) [order 2] : {fs_ch = int32(0);}
    (junction 190) -> (junction 192) : {fs_ch = RC_MAP_FAILSAFE;}
    (junction 192) -> (junction 191)
    (junction 191) -> (junction 193)
    (junction 193) -> (junction 194) [order 1] : [RC_FAILS_THR > 0 && fs_ch > 0]
    (junction 194) -> (junction 195) : [RC_FAILS_THR < RC_MIN(fs_ch) &&  input_rc.values(fs_ch) < RC_FAILS_THR || ...
        | RC_FAILS_THR > RC_MAX(fs_ch) && input_rc.values(fs_ch) > RC_FAILS_THR]
    (junction 195) -> (junction 197) : {signal_lost = true;}
    (junction 193) -> (junction 196) [order 2]
    (junction 197) -> (junction 196)
    (junction 196) -> (junction 198)
  (default) -> (junction 249)
  (junction 249) -> (junction 248) : {signal_lost=true;}
  (junction 248) -> (junction 211) [order 1] : [input_rc.rc_lost || input_rc.rc_failsafe || input_rc.channel_count < 4]
  (junction 248) -> (junction 242) [order 2]
  (junction 211) -> (junction 212) : {signal_lost = true;}
  (junction 242) -> (junction 250) [order 1] : [(input_rc.input_source == INPUT_RC.RC_INPUT_SOURCE_PX4FMU_PPM || ...
      | input_rc.input_source == INPUT_RC.RC_INPUT_SOURCE_PX4IO_PPM)&& ...
      | input_rc.channel_count == 16]
  (junction 242) -> (junction 239) [order 2] : {failsafe_rc_lost_check();}
  (junction 250) -> (junction 244) : {rfd_rc_lost_check();}
  (junction 244) -> (junction 239)
  (junction 212) -> (junction 244)
  (junction 239) -> (junction 247)
  data: input_rc input; signal_lost output; RC_MAP_FAILSAFE parameter; RC_FAILS_THR parameter; RC_MIN data_store_memory; RC_MAX data_store_memory

== matlab function rc_update/Handle Rc_Value/RC Function/MATLAB Function ==
  data: channel output int8 size=6; RC_MAP_FLTM_BTN parameter
function channel = map_flight_modes_buttons(RC_MAP_FLTM_BTN)
channel = -ones(6,1, 'int8');
k = 1;
for i = 1:18
    if bitget(RC_MAP_FLTM_BTN, i) > 0
        channel(k) = int8(i - 1);
        k = k + 1;
    end
    if k > 6
        break;
    end
end

== matlab function rc_update/Manual Switches/MATLAB Function ==
  data: rc_values input; mode_slot output; channel input
function mode_slot = get_mode_slot(rc_values, channel)


mode_slot = uint8(0);

if channel > 0
    num_slots = uint8(MANUAL_CONTROL_SWITCHES.MODE_SLOT_NUM);
    slot_width_half  = single(1) / single(num_slots);
    slot_min = single(-1.05);
    slot_max = single(1.05);
    value = rc_values(channel);
    tmp = floor((((((value - slot_min) * single(num_slots)) + slot_width_half) / (slot_max - slot_min)) + slot_width_half) + 1.0);
    mode_slot = min(num_slots, uint8(tmp));
end

== matlab function rc_update/Manual Switches/For Each Subsystem/MATLAB Function1 ==
  data: rc_values input; switches output; channel input; threshold input
function switches = get_rc_sw2pos_position(rc_values, channel, threshold )

if channel > 0
    value = rc_values(channel) * 0.5 + 0.5;

    if abs(value) > abs(threshold)
        switches = uint8(1);  % SWITCH_POS_ON
    else
        switches = uint8(3); % SWITCH_POS_OFF
    end
else
    switches = uint8(0); % SWITCH_POS_NONE
end

== matlab function rc_update/Manual Setpoint/For Each Subsystem/MATLAB Function ==
  data: rc_values input; stick output; channel input
function stick = get_rc_value(rc_values, channel)

stick = single(0);

if channel > 0
    stick = rc_values(channel);
end
